simulink model "linear_model_p2"  (R2022a)
settings: Solver=VariableStepAuto  StartTime=0.0  StopTime=5  RelTol=1e-4
libraries: slpidlib x1
settings Model: Creator=ASUS  LastModifiedBy=ASUS

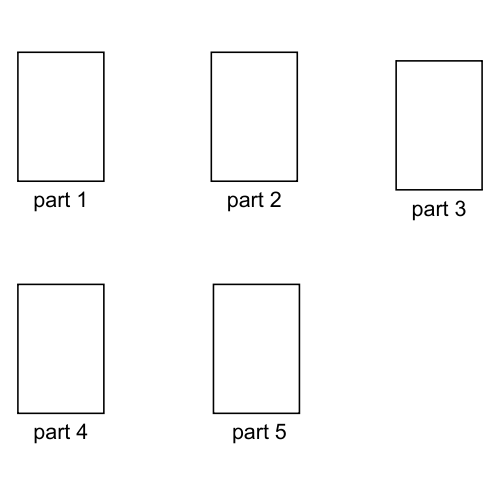
[thumbnail: Simulink's stored preview of the top-level diagram]
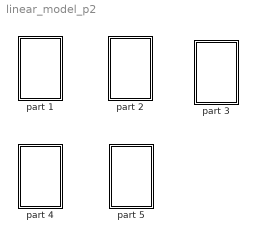
== system linear_model_p2 ==
  " part 5" : Subsystem
  part 1 : Subsystem
  part 2 : Subsystem
  part 3 : Subsystem
  part 4 : Subsystem

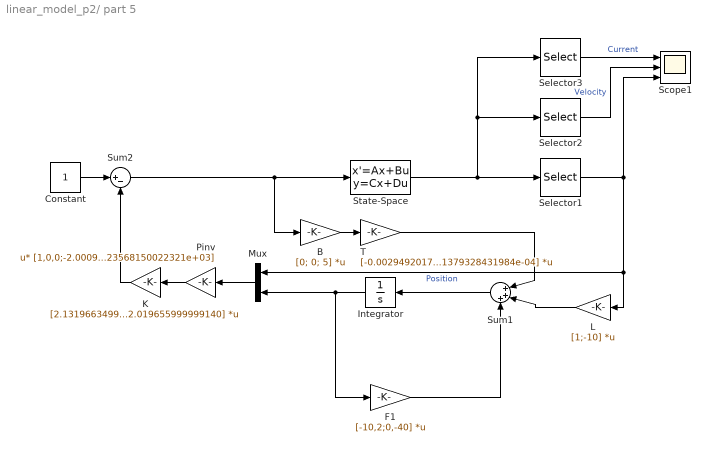
== system linear_model_p2/ part 5 ==
  B : Gain  Gain=[0; 0; 5]  Multiplication=Matrix(K*u)
  Constant : Constant
  F1 : Gain  Gain=[-10,2;0,-40]  Multiplication=Matrix(K*u)
  Integrator : Integrator
  K : Gain  Gain=[2.131966349959954e+03,89.493722718849200,-12.019655999999140]  Multiplication=Matrix(K*u)
  L : Gain  Gain=[1;-10]  Multiplication=Matrix(K*u)
  Mux : Mux  Inputs=2
  Pinv : Gain  Gain=[1,0,0;-2.000982800000000e+02,3.499507200000001e+03,-7.125666799999996e+02;1.875279059383836e+03,-2.734396904301236e+04,6.623568150022321e+03]  Multiplication=Matrix(u*K)
  Scope1 : Scope  NumInputPorts=3
  Selector1 : Selector  InputPortWidth=3  IndexOptions=Index vector (dialog)  Indices=[1]  OutputSizes=1
  Selector2 : Selector  InputPortWidth=3  IndexOptions=Index vector (dialog)  Indices=[2]  OutputSizes=1
  Selector3 : Selector  InputPortWidth=3  IndexOptions=Index vector (dialog)  Indices=[3]  OutputSizes=1
  State-Space : StateSpace  A=[0 1 0;224.83 -0.09828 26.867;0 0 -250]  B=[0;0;5]  C=[1 0 0;0 1 0;0 0 1]  D=[0;0;0]  InitialCondition=0  ContinuousStateAttributes={'Position','Velocity','Current'}
  Sum1 : Sum  Inputs=|+++
  Sum2 : Sum  Inputs=|+-
  T : Gain  Gain=[-0.002949201780729,0.001792661734103,1.928554204169491e-04;-0.295297322723415,0.007400616382537,9.471379328431984e-04]  Multiplication=Matrix(K*u)
  wires:
  Integrator/1 -> Mux/2, F1/1
  Sum2/1 -> B/1, State-Space/1
  Sum1/1 -> Integrator/1
  Selector1/1 -> Scope1/3, L/1, Mux/1  "Position"
  Selector2/1 -> Scope1/2  "Velocity"
  Selector3/1 -> Scope1/1  "Current"
  Constant/1 -> Sum2/1
  K/1 -> Sum2/2
  L/1 -> Sum1/2
  State-Space/1 -> Selector2/1, Selector3/1, Selector1/1
  T/1 -> Sum1/1
  F1/1 -> Sum1/3
  Pinv/1 -> K/1
  Mux/1 -> Pinv/1
  B/1 -> T/1

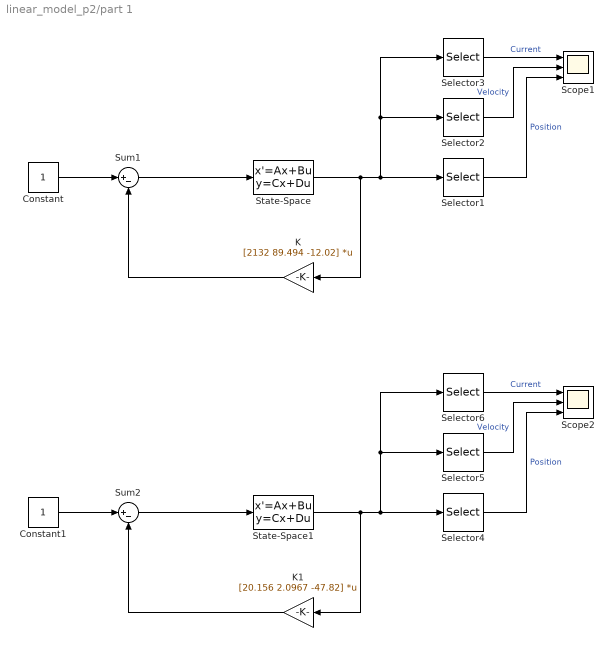
== system linear_model_p2/part 1 ==
  Constant : Constant
  Constant1 : Constant
  K : Gain  Gain=[2132 89.494 -12.02]  Multiplication=Matrix(K*u)
  K1 : Gain  Gain=[20.156 2.0967 -47.82]  Multiplication=Matrix(K*u)
  Scope1 : Scope  NumInputPorts=3
  Scope2 : Scope  NumInputPorts=3
  Selector1 : Selector  InputPortWidth=3  IndexOptions=Index vector (dialog)  Indices=[1]  OutputSizes=1
  Selector2 : Selector  InputPortWidth=3  IndexOptions=Index vector (dialog)  Indices=[2]  OutputSizes=1
  Selector3 : Selector  InputPortWidth=3  IndexOptions=Index vector (dialog)  Indices=[3]  OutputSizes=1
  Selector4 : Selector  InputPortWidth=3  IndexOptions=Index vector (dialog)  Indices=[1]  OutputSizes=1
  Selector5 : Selector  InputPortWidth=3  IndexOptions=Index vector (dialog)  Indices=[2]  OutputSizes=1
  Selector6 : Selector  InputPortWidth=3  IndexOptions=Index vector (dialog)  Indices=[3]  OutputSizes=1
  State-Space : StateSpace  A=[0 1 0;224.83 -0.09828 26.867;0 0 -250]  B=[0;0;5]  C=[1 0 0;0 1 0;0 0 1]  D=[0;0;0]  InitialCondition=0  ContinuousStateAttributes={'Position','Velocity','Current'}
  State-Space1 : StateSpace  A=[0 1 0;224.83 -0.09828 26.867;0 0 -250]  B=[0;0;5]  C=[1 0 0;0 1 0;0 0 1]  D=[0;0;0]  InitialCondition=0  ContinuousStateAttributes={'Position','Velocity','Current'}
  Sum1 : Sum  Inputs=|+-
  Sum2 : Sum  Inputs=|+-
  wires:
  State-Space/1 -> Selector2/1, Selector3/1, Selector1/1, K/1
  Selector6/1 -> Scope2/1  "Current"
  Constant/1 -> Sum1/1
  Sum1/1 -> State-Space/1
  Selector3/1 -> Scope1/1  "Current"
  State-Space1/1 -> Selector5/1, Selector6/1, Selector4/1, K1/1
  Selector1/1 -> Scope1/3  "Position"
  Selector2/1 -> Scope1/2  "Velocity"
  Sum2/1 -> State-Space1/1
  K1/1 -> Sum2/2
  Selector5/1 -> Scope2/2  "Velocity"
  Selector4/1 -> Scope2/3  "Position"
  K/1 -> Sum1/2
  Constant1/1 -> Sum2/1

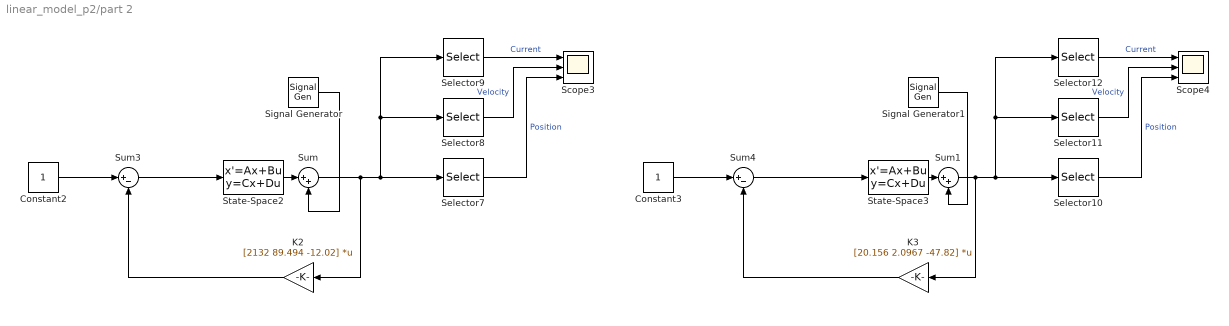
== system linear_model_p2/part 2 ==
  Constant2 : Constant
  Constant3 : Constant
  K2 : Gain  Gain=[2132 89.494 -12.02]  Multiplication=Matrix(K*u)
  K3 : Gain  Gain=[20.156 2.0967 -47.82]  Multiplication=Matrix(K*u)
  Scope3 : Scope  NumInputPorts=3
  Scope4 : Scope  NumInputPorts=3
  Selector10 : Selector  InputPortWidth=3  IndexOptions=Index vector (dialog)  Indices=[1]  OutputSizes=1
  Selector11 : Selector  InputPortWidth=3  IndexOptions=Index vector (dialog)  Indices=[2]  OutputSizes=1
  Selector12 : Selector  InputPortWidth=3  IndexOptions=Index vector (dialog)  Indices=[3]  OutputSizes=1
  Selector7 : Selector  InputPortWidth=3  IndexOptions=Index vector (dialog)  Indices=[1]  OutputSizes=1
  Selector8 : Selector  InputPortWidth=3  IndexOptions=Index vector (dialog)  Indices=[2]  OutputSizes=1
  Selector9 : Selector  InputPortWidth=3  IndexOptions=Index vector (dialog)  Indices=[3]  OutputSizes=1
  Signal Generator : SignalGenerator  Amplitude=0.05  Frequency=5  Units=rad/sec
  Signal Generator1 : SignalGenerator  Amplitude=0.05  Frequency=5  Units=rad/sec
  State-Space2 : StateSpace  A=[0 1 0;224.83 -0.09828 26.867;0 0 -250]  B=[0;0;5]  C=[1 0 0;0 1 0;0 0 1]  D=[0;0;0]  InitialCondition=0  ContinuousStateAttributes={'Position','Velocity','Current'}
  State-Space3 : StateSpace  A=[0 1 0;224.83 -0.09828 26.867;0 0 -250]  B=[0;0;5]  C=[1 0 0;0 1 0;0 0 1]  D=[0;0;0]  InitialCondition=0  ContinuousStateAttributes={'Position','Velocity','Current'}
  Sum : Sum  Inputs=|++
  Sum1 : Sum  Inputs=|++
  Sum3 : Sum  Inputs=|+-
  Sum4 : Sum  Inputs=|+-
  wires:
  Selector11/1 -> Scope4/2  "Velocity"
  K2/1 -> Sum3/2
  Sum1/1 -> Selector11/1, Selector12/1, Selector10/1, K3/1
  Selector10/1 -> Scope4/3  "Position"
  Sum/1 -> Selector8/1, Selector9/1, Selector7/1, K2/1
  Constant3/1 -> Sum4/1
  Selector12/1 -> Scope4/1  "Current"
  Sum3/1 -> State-Space2/1
  K3/1 -> Sum4/2
  Sum4/1 -> State-Space3/1
  Constant2/1 -> Sum3/1
  Selector9/1 -> Scope3/1  "Current"
  Selector8/1 -> Scope3/2  "Velocity"
  Selector7/1 -> Scope3/3  "Position"
  Signal Generator/1 -> Sum/2
  State-Space2/1 -> Sum/1
  Signal Generator1/1 -> Sum1/2
  State-Space3/1 -> Sum1/1

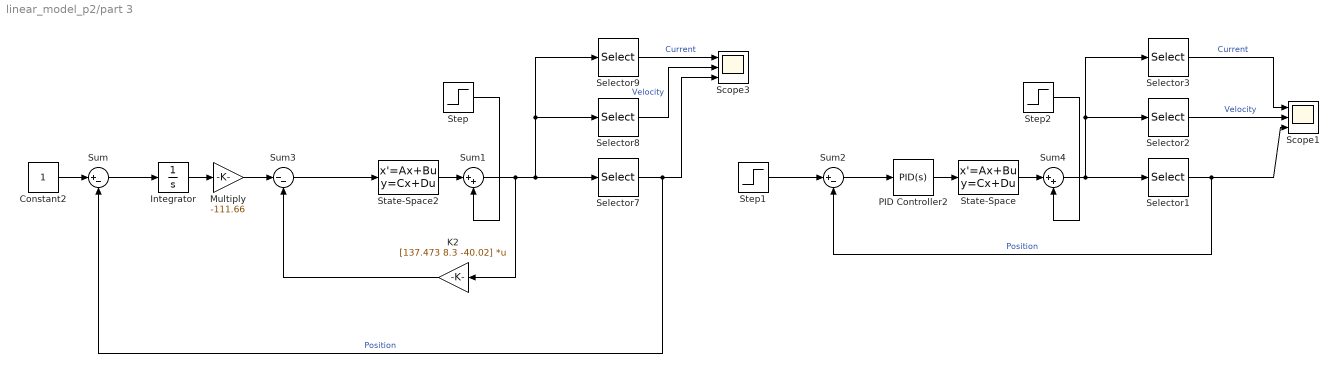
== system linear_model_p2/part 3 ==
  Constant2 : Constant
  Integrator : Integrator
  K2 : Gain  Gain=[137.473 8.3 -40.02]  Multiplication=Matrix(K*u)
  Multiply : Gain  Gain=-111.66
  PID Controller2 : slpidlib/PID Controller  Controller=PID  Form=Parallel  TimeDomain=Continuous-time  UseExternalTs=off  SampleTime=-1  IntegratorMethod=Forward Euler  FilterMethod=Forward Euler  ControllerParametersSource=internal  P=1000  I=1000  UseKiTs=off  D=150  N=1000  UseFilter=on  TunerSelectOption=Transfer Function Based (PID Tuner App)  InitialConditionSource=internal  InitialConditionForIntegrator=0  InitialConditionForFilter=0  DifferentiatorICPrevScaledInput=0  ExternalReset=none  TrackingMode=off  Kt=1  LimitOutput=off  SatLimitsSource=internal  UpperSaturationLimit=inf  LowerSaturationLimit=-inf  LinearizeAsGain=on  AntiWindupMode=none  Kb=1  POutMin=[]  POutMax=[]  IOutMin=[]  IOutMax=[]  DOutMin=[]  DOutMax=[]  NOutMin=[]  NOutMax=[]  SumOutMin=[]  SumOutMax=[]  SaturationOutMin=[]  SaturationOutMax=[]  PParamMin=[]  PParamMax=[]  IParamMin=[]  IParamMax=[]  DParamMin=[]  DParamMax=[]  NParamMin=[]  NParamMax=[]  KbParamMin=[]  KbParamMax=[]  KtParamMin=[]  KtParamMax=[]  KbOutMin=[]  KbOutMax=[]  KtOutMin=[]  KtOutMax=[]  IntegratorOutMin=[]  IntegratorOutMax=[]  FilterOutMin=[]  FilterOutMax=[]  SumI1OutMin=[]  SumI1OutMax=[]  SumI2OutMin=[]  SumI2OutMax=[]  SumI3OutMin=[]  SumI3OutMax=[]  SumI4OutMin=[]  SumI4OutMax=[]  SumDOutMin=[]  SumDOutMax=[]  DifferentiatorOutMin=[]  DifferentiatorOutMax=[]  FilterDiffOutCoefMin=[]  FilterDiffOutCoefMax=[]  ReciprocalOutMin=[]  ReciprocalOutMax=[]  SumDenOutMin=[]  SumDenOutMax=[]  SumNumOutMin=[]  SumNumOutMax=[]  DivideOutMin=[]  DivideOutMax=[]  UdiffTsProdOutMin=[]  UdiffTsProdOutMax=[]  NTsProdOutMin=[]  NTsProdOutMax=[]  UintegralTsProdOutMin=[]  UintegralTsProdOutMax=[]  UngainTsProdOutMin=[]  UngainTsProdOutMax=[]  IntegratorContinuousStateAttributes=''  IntegratorStateMustResolveToSignalObject=off  IntegratorRTWStateStorageClass=Auto  FilterContinuousStateAttributes=''  FilterStateMustResolveToSignalObject=off  FilterRTWStateStorageClass=Auto  ParallelPVariant=InternalParameters  IdealPVariant=Disabled  IVariant=InternalParameters  DVariant=InternalParameters  IntegratorVariant=Continuous  SatVariant=Disabled  AWVariant=Passthrough  PCopyVariant=Disabled  TRVariant=Disabled  FdbkBlocksVariant=Forward  IdealPFdbkVariant=Disabled  SatFdbkVariant=Disabled  DerivativeFilterVariant=ContFilter  NVariant=InternalParameters  NCopyVariant=Disabled  FilterICVariant=InternalICsFilter  IntegratorICVariant=InternalICs  ExternalResetVariant=Disabled  TRSumVariant=Passthrough  SumFdbkVariant=Disabled  SumVariant=Sum_PID  TsampFilterVariant=InternalTs  TsampNgainVariant=Passthrough  TsampIntegralVariant=Passthrough  ExternalSaturationOutDataTypeStr=Inherit: Same as second input  aMode=0
  Scope1 : Scope  NumInputPorts=3
  Scope3 : Scope  NumInputPorts=3
  Selector1 : Selector  InputPortWidth=3  IndexOptions=Index vector (dialog)  Indices=[1]  OutputSizes=1
  Selector2 : Selector  InputPortWidth=3  IndexOptions=Index vector (dialog)  Indices=[2]  OutputSizes=1
  Selector3 : Selector  InputPortWidth=3  IndexOptions=Index vector (dialog)  Indices=[3]  OutputSizes=1
  Selector7 : Selector  InputPortWidth=3  IndexOptions=Index vector (dialog)  Indices=[1]  OutputSizes=1
  Selector8 : Selector  InputPortWidth=3  IndexOptions=Index vector (dialog)  Indices=[2]  OutputSizes=1
  Selector9 : Selector  InputPortWidth=3  IndexOptions=Index vector (dialog)  Indices=[3]  OutputSizes=1
  State-Space : StateSpace  A=[0 1 0;224.83 -0.09828 26.867;0 0 -250]  B=[0;0;5]  C=[1 0 0;0 1 0;0 0 1]  D=[0;0;0]  InitialCondition=0  ContinuousStateAttributes={'Position','Velocity','Current'}
  State-Space2 : StateSpace  A=[0 1 0;224.83 -0.09828 26.867;0 0 -250]  B=[0;0;5]  C=[1 0 0;0 1 0;0 0 1]  D=[0;0;0]  InitialCondition=0  ContinuousStateAttributes={'Position','Velocity','Current'}
  Step : Step  Time=0  After=5  SampleTime=0
  Step1 : Step  Time=0  SampleTime=0
  Step2 : Step  Time=0  After=5  SampleTime=0
  Sum : Sum  Inputs=|+-
  Sum1 : Sum  Inputs=|++
  Sum2 : Sum  Inputs=|+-
  Sum3 : Sum  Inputs=|--
  Sum4 : Sum  Inputs=|++
  wires:
  K2/1 -> Sum3/2
  Sum1/1 -> Selector8/1, Selector9/1, Selector7/1, K2/1
  Selector9/1 -> Scope3/1  "Current"
  Sum3/1 -> State-Space2/1
  Selector8/1 -> Scope3/2  "Velocity"
  Selector7/1 -> Scope3/3, Sum/2  "Position"
  Integrator/1 -> Multiply/1
  Multiply/1 -> Sum3/1
  Sum/1 -> Integrator/1
  Constant2/1 -> Sum/1
  State-Space2/1 -> Sum1/1
  Step/1 -> Sum1/2
  Sum4/1 -> Selector2/1, Selector3/1, Selector1/1
  Selector2/1 -> Scope1/2  "Velocity"
  Selector3/1 -> Scope1/1  "Current"
  PID Controller2/1 -> State-Space/1
  Selector1/1 -> Scope1/3, Sum2/2  "Position"
  Sum2/1 -> PID Controller2/1
  Step1/1 -> Sum2/1
  Step2/1 -> Sum4/2
  State-Space/1 -> Sum4/1

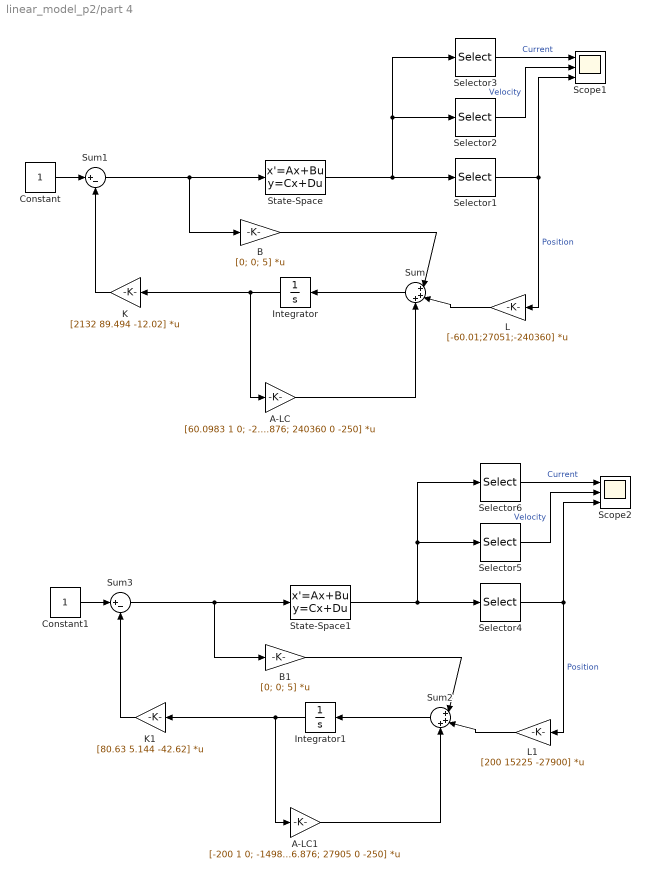
== system linear_model_p2/part 4 ==
  A-LC : Gain  Gain=[60.0983 1 0; -26806 -0.0983 26.876; 240360 0 -250]  Multiplication=Matrix(K*u)
  A-LC1 : Gain  Gain=|  Multiplication=Matrix(K*u)
      | [-200 1 0;
      | -14980 -0.09828 26.876;
      | 27905 0 -250]
  B : Gain  Gain=[0; 0; 5]  Multiplication=Matrix(K*u)
  B1 : Gain  Gain=[0; 0; 5]  Multiplication=Matrix(K*u)
  Constant : Constant
  Constant1 : Constant
  Integrator : Integrator
  Integrator1 : Integrator
  K : Gain  Gain=[2132 89.494 -12.02]  Multiplication=Matrix(K*u)
  K1 : Gain  Gain=[80.63 5.144 -42.62]  Multiplication=Matrix(K*u)
  L : Gain  Gain=[-60.01;27051;-240360]  Multiplication=Matrix(K*u)
  L1 : Gain  Gain=|  Multiplication=Matrix(K*u)
      | [200
      | 15225
      | -27900]
  Scope1 : Scope  NumInputPorts=3
  Scope2 : Scope  NumInputPorts=3
  Selector1 : Selector  InputPortWidth=3  IndexOptions=Index vector (dialog)  Indices=[1]  OutputSizes=1
  Selector2 : Selector  InputPortWidth=3  IndexOptions=Index vector (dialog)  Indices=[2]  OutputSizes=1
  Selector3 : Selector  InputPortWidth=3  IndexOptions=Index vector (dialog)  Indices=[3]  OutputSizes=1
  Selector4 : Selector  InputPortWidth=3  IndexOptions=Index vector (dialog)  Indices=[1]  OutputSizes=1
  Selector5 : Selector  InputPortWidth=3  IndexOptions=Index vector (dialog)  Indices=[2]  OutputSizes=1
  Selector6 : Selector  InputPortWidth=3  IndexOptions=Index vector (dialog)  Indices=[3]  OutputSizes=1
  State-Space : StateSpace  A=[0 1 0;224.83 -0.09828 26.867;0 0 -250]  B=[0;0;5]  C=[1 0 0;0 1 0;0 0 1]  D=[0;0;0]  InitialCondition=0  ContinuousStateAttributes={'Position','Velocity','Current'}
  State-Space1 : StateSpace  A=[0 1 0;224.83 -0.09828 26.867;0 0 -250]  B=[0;0;5]  C=[1 0 0;0 1 0;0 0 1]  D=[0;0;0]  InitialCondition=0  ContinuousStateAttributes={'Position','Velocity','Current'}
  Sum : Sum  Inputs=|+++
  Sum1 : Sum  Inputs=|+-
  Sum2 : Sum  Inputs=|+++
  Sum3 : Sum  Inputs=|+-
  wires:
  Selector1/1 -> Scope1/3, L/1  "Position"
  Selector2/1 -> Scope1/2  "Velocity"
  Sum1/1 -> B/1, State-Space/1
  K/1 -> Sum1/2
  Constant/1 -> Sum1/1
  Selector3/1 -> Scope1/1  "Current"
  State-Space/1 -> Selector2/1, Selector3/1, Selector1/1
  L/1 -> Sum/2
  B/1 -> Sum/1
  A-LC/1 -> Sum/3
  Sum/1 -> Integrator/1
  Integrator/1 -> A-LC/1, K/1
  State-Space1/1 -> Selector5/1, Selector6/1, Selector4/1
  Constant1/1 -> Sum3/1
  B1/1 -> Sum2/1
  Integrator1/1 -> A-LC1/1, K1/1
  Sum3/1 -> B1/1, State-Space1/1
  Sum2/1 -> Integrator1/1
  A-LC1/1 -> Sum2/3
  Selector6/1 -> Scope2/1  "Current"
  L1/1 -> Sum2/2
  Selector4/1 -> Scope2/3, L1/1  "Position"
  K1/1 -> Sum3/2
  Selector5/1 -> Scope2/2  "Velocity"
